simulink model "PitchSys"  (Simulink 10.3)
settings: Solver=ode1  StartTime=0.00  StopTime=10.00  FixedStep=0.01  RelTol=1e-3  EnableMultiTasking=on
values from neighbouring files (symbols this model uses):
  Jp = 2*m1*(l2^2)    (= 0.0004949)    [heli.m]
  k_d = 1.5    [heli.m]
  k_s = 4    [heli.m]
  l2 = 0.070    (= 0.07)    [heli.m]
settings Model: Creator=bjones  LastModifiedBy=seb  MultithreadedSim=on
settings OptimizationCC: BlockReduction=off  BooleanDataType=off
settings DebuggingCC: SaveWithParameterizedLinksMsg=none  SignalResolutionControl=TryResolveAllWithWarning  MultiTaskDSMMsg=warning  MultiTaskCondExecSysMsg=none
settings HardwareCC: TargetUnknown=on
settings ConfigComp: CovSFcnEnable=off

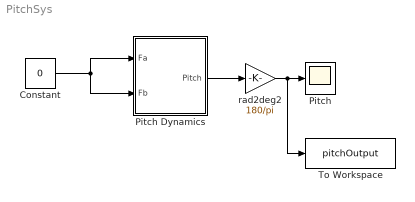
== system PitchSys ==
  Constant : Constant  Value=0
  Pitch : Scope
  Pitch Dynamics : Subsystem
  To Workspace : ToWorkspace  VariableName=pitchOutput  SaveFormat=Timeseries  SampleTime=-1
  rad2deg2 : Gain  Gain=180/pi  SaturateOnIntegerOverflow=on  OutDataTypeStr=Inherit: Same as input  ParamDataTypeStr=Inherit: Same as input
  wires:
  Pitch Dynamics/1(Pitch) -> rad2deg2/1
  rad2deg2/1 -> To Workspace/1, Pitch/1
  Constant/1 -> Pitch Dynamics/1(Fa), Pitch Dynamics/2(Fb)

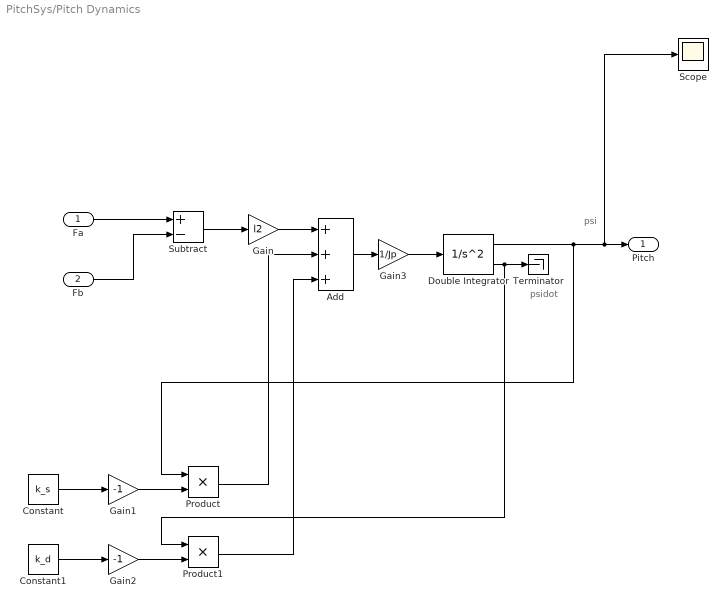
== system PitchSys/Pitch Dynamics ==
  note: psi
  note: psidot
  Fa : Inport
  Fb : Inport  Port=2
  Add : Sum  Inputs=+++
  Constant : Constant  Value=k_s
  Constant1 : Constant  Value=k_d
  Double Integrator : SecondOrderIntegrator  ICX=p_lim_u  LimitX=on  UpperLimitX=p_lim_u  LowerLimitX=p_lim_l
  Gain : Gain  Gain=l2
  Gain1 : Gain  Gain=-1
  Gain2 : Gain  Gain=-1
  Gain3 : Gain  Gain=1/Jp
  Product : Product
  Product1 : Product
  Scope : Scope
  Subtract : Sum  Inputs=+-
  Terminator : Terminator
  Pitch : Outport
  wires:
  Double Integrator/1 -> Product/1, Scope/1, Pitch/1
  Double Integrator/2 -> Product1/1, Terminator/1
  Fa/1 -> Subtract/1
  Fb/1 -> Subtract/2
  Subtract/1 -> Gain/1
  Gain/1 -> Add/1
  Gain1/1 -> Product/2
  Gain2/1 -> Product1/2
  Product/1 -> Add/2
  Product1/1 -> Add/3
  Constant/1 -> Gain1/1
  Constant1/1 -> Gain2/1
  Add/1 -> Gain3/1
  Gain3/1 -> Double Integrator/1
